simulink model "pendulum_DRF"  (R2019b)
settings: Solver=VariableStepAuto  StartTime=0.0  StopTime=20  RelTol=1e-3
values from neighbouring files (symbols this model uses):
  b = 0.3    [pendulum_DRF_design.m]
  D = 0.5    [pendulum_DRF_design.m]
  f_disturb = 2    [pendulum_DRF_design.m]
  g = 9.81    [pendulum_DRF_design.m]
  G__DRF = ( (s^2)/wz^2 + 1 )/( s^2/wp^2 + 1)    [notch_filter.m]    (also in pendulum_DRF_design.m = ( s^2/wz^2 +  1 )/( s^2/wp^2 +  1))
  I = 1    [pendulum_DRF_design.m]
  l = 0.1    [pendulum_DRF_design.m]
  m = 1    [pendulum_DRF_design.m]
  P = 3    [pendulum_DRF_design.m]
libraries: simulink x1
settings Model: Creator=henry  LastModifiedBy=henry

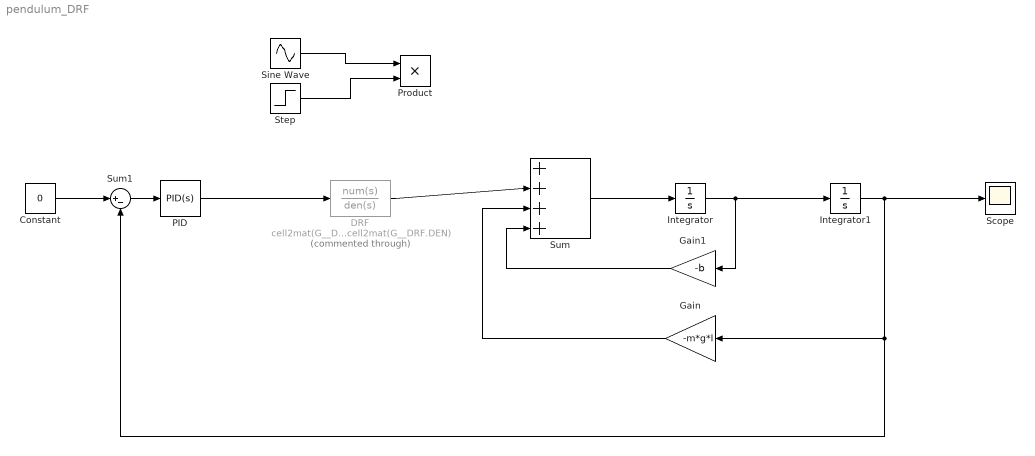
== system pendulum_DRF ==
  Constant : Constant  Value=0
  DRF : TransferFcn  Commented=through  Numerator=cell2mat(G__DRF.NUM)  Denominator=cell2mat(G__DRF.DEN)
  Gain : Gain  Gain=-m*g*l
  Gain1 : Gain  Gain=-b
  Integrator : Integrator
  Integrator1 : Integrator  InitialCondition=-pi/4
  PID : simulink/Continuous/PID Controller  Controller=PID  Form=Parallel  TimeDomain=Continuous-time  SampleTime=-1  IntegratorMethod=Forward Euler  FilterMethod=Forward Euler  ControllerParametersSource=internal  P=P  I=I  D=D  UseFilter=on  N=100  TunerSelectOption=Transfer Function Based (PID Tuner App)  InitialConditionSource=internal  InitialConditionForIntegrator=0  InitialConditionForFilter=0  DifferentiatorICPrevScaledInput=0  ExternalReset=none  TrackingMode=off  Kt=1  LimitOutput=off  UpperSaturationLimit=inf  LowerSaturationLimit=-inf  LinearizeAsGain=on  AntiWindupMode=none  Kb=1  POutMin=[]  POutMax=[]  IOutMin=[]  IOutMax=[]  DOutMin=[]  DOutMax=[]  NOutMin=[]  NOutMax=[]  SumOutMin=[]  SumOutMax=[]  SaturationOutMin=[]  SaturationOutMax=[]  PParamMin=[]  PParamMax=[]  IParamMin=[]  IParamMax=[]  DParamMin=[]  DParamMax=[]  NParamMin=[]  NParamMax=[]  KbParamMin=[]  KbParamMax=[]  KtParamMin=[]  KtParamMax=[]  KbOutMin=[]  KbOutMax=[]  KtOutMin=[]  KtOutMax=[]  IntegratorOutMin=[]  IntegratorOutMax=[]  FilterOutMin=[]  FilterOutMax=[]  SumI1OutMin=[]  SumI1OutMax=[]  SumI2OutMin=[]  SumI2OutMax=[]  SumI3OutMin=[]  SumI3OutMax=[]  SumI4OutMin=[]  SumI4OutMax=[]  SumDOutMin=[]  SumDOutMax=[]  DifferentiatorOutMin=[]  DifferentiatorOutMax=[]  FilterDiffOutCoefMin=[]  FilterDiffOutCoefMax=[]  ReciprocalOutMin=[]  ReciprocalOutMax=[]  SumDenOutMin=[]  SumDenOutMax=[]  SumNumOutMin=[]  SumNumOutMax=[]  DivideOutMin=[]  DivideOutMax=[]  IntegratorContinuousStateAttributes=''  IntegratorStateMustResolveToSignalObject=off  IntegratorRTWStateStorageClass=Auto  FilterContinuousStateAttributes=''  FilterStateMustResolveToSignalObject=off  FilterRTWStateStorageClass=Auto  ParallelPVariant=InternalParameters  IdealPVariant=Disabled  IVariant=InternalParameters  DVariant=InternalParameters  IntegratorVariant=Continuous  SatVariant=Disabled  AWVariant=Passthrough  PCopyVariant=Disabled  TRVariant=Disabled  FdbkBlocksVariant=Forward  IdealPFdbkVariant=Disabled  SatFdbkVariant=Disabled  DerivativeFilterVariant=ContFilter  NVariant=InternalParameters  NCopyVariant=Disabled  FilterICVariant=InternalICsFilter  IntegratorICVariant=InternalICs  ExternalResetVariant=Disabled  TRSumVariant=Passthrough  SumFdbkVariant=Disabled  SumVariant=Sum_PID
  Product : Product
  Scope : Scope
  Sine Wave : Sin  Amplitude=5  Frequency=f_disturb  SampleTime=0
  Step : Step  Time=10  SampleTime=0
  Sum : Sum  Inputs=|++++
  Sum1 : Sum  Inputs=|+-
  wires:
  Integrator/1 -> Gain1/1, Integrator1/1
  Sum/1 -> Integrator/1
  Integrator1/1 -> Gain/1, Sum1/2, Scope/1
  Gain/1 -> Sum/3
  Gain1/1 -> Sum/4
  Constant/1 -> Sum1/1
  Sum1/1 -> PID/1
  DRF/1 -> Sum/2
  PID/1 -> DRF/1
  Step/1 -> Product/2
  Sine Wave/1 -> Product/1
